simulink model "rev0BB"  (R2017b)
settings: Solver=FixedStepDiscrete  StartTime=0  StopTime=(((preLen+100+dataLenSymbols)*1+pad_first*3)*basePer)  RelTol=1e-3
values from neighbouring files (symbols this model uses):
  ack_stf_len_symbols = length(x_ACK_STF)    [rev0BB_setup.m]
  agc_delay_lag = 32    [rev0BB_setup.m]
  agc_detector_coef = ones(1,agc_detector_taps)./agc_detector_taps    [rev0BB_setup.m]
  agc_on = true    [rev0BB_startup.m]
  agc_sat_low = -agcSaturation    (= -12)    [rev0BB_setup.m]
  agc_sat_up = agcSaturation    (= 12)    [rev0BB_setup.m]
  agcDesired = 0    [rev0BB_setup.m]
  agcExpDomain = agcSaturation    (= 12)    [rev0BB_setup.m]
  agcExpResolution = 2^-5    (= 0.03125)    [rev0BB_setup.m]
  agcPwrAvgNum = 128    [rev0BB_setup.m]
  agcSaturation = 12    [rev0BB_setup.m]
  agcSettleThresh = 0.65    [rev0BB_setup.m]
  agcStep = 2^-8    (= 0.00390625)    [rev0BB_setup.m]
  atanDomain = 5    [rev0BB_setup.m]
  atanDomainTiming = 256    [rev0BB_setup.m]
  atanResolution = 2^-9    (= 0.001953125)    [rev0BB_setup.m]
  atanResolutionTiming = 2^-5    (= 0.03125)    [rev0BB_setup.m]
  averaging_num = ones(1, averaging_samples)    [rev0BB_setup.m]
  averaging_samples = 128    [rev0BB_setup.m]
  awgnSeed = abs(dBSnrRange(dBSnrInd)*1000+trial+10000000)    [plotBer.m]    (also in rev0BB_startup.m = 67)
  basePer = 1/baseFreq    (= 5e-08)    [rev0BB_setup.m]
  bitsPerSymbolHeader = log2(radixHeader)    [rev0BB_setup.m]
  bitsPerSymbolMax = log2(radixMax)    [rev0BB_setup.m]
  cal_sig_i_mult = 1.0    (= 1)    [rev0BB_startup.m]
  cal_sig_i_offset = 0.0    (= 0)    [rev0BB_startup.m]
  cal_sig_q_mult = 1.0    (= 1)    [rev0BB_startup.m]
  cal_sig_q_offset = 0.0    (= 0)    [rev0BB_startup.m]
  cefEarlyWarning = 256    [rev0BB_setup.m]
  cefLen = length(x_CEF)    [rev0BB_setup.m]
  channelFIR = zeros(1, round(maxSampleDelay)+1)    [rev0BB_startup.m]
  coarseCFOAdaptDelay = 1    [rev0BB_setup.m]
  cr_i = 0.020    (= 0.02)    [rev0BB_setup.m]
  cr_i_preamp = 2^-9    (= 0.001953125)    [rev0BB_setup.m]
  cr_int1_sat_low = -cr_integrator1_saturation    (= -0.6)    [rev0BB_setup.m]
  cr_int1_sat_up = cr_integrator1_saturation    (= 0.6)    [rev0BB_setup.m]
  cr_integrator1_decay = 1    [rev0BB_setup.m]
  cr_integrator1_saturation = 0.6    [rev0BB_setup.m]
  cr_mult_pipeline = 0    [rev0BB_setup.m]
  cr_p = 0.015    [rev0BB_setup.m]
  cr_sat2_low = -cr_saturation2    (= -0.6)    [rev0BB_setup.m]
  cr_sat2_up = cr_saturation2    (= 0.6)    [rev0BB_setup.m]
  cr_smooth_num = (1/cr_smooth_samples).*ones(1, cr_smooth_samples)    [rev0BB_setup.m]
  D_128 = [ 1,  8,  2,  4, 16, 32, 64]    [golay.m]    (also in rev0BB_setup.m)
  D_32 = [ 1,  4,  8,  2, 16]    [golay.m]    (also in rev0BB_setup.m)
  dataLenSymbols = header_len_bytes*8/bitsPerSymbolHeader + frame_len_bytes*8/bitsPerSymbol    [rev0BB_setup.m]
  default_channel = 3    [rev0BB_setup.m]
  dmm_coefs = ones(1,dmm_samples)./dmm_samples    [rev0BB_setup.m]
  dst_field_len = 8    [rev0BB_setup.m]
  expDomain = 3.3    [rev0BB_setup.m]
  expResolution = 2^-5    (= 0.03125)    [rev0BB_setup.m]
  expTol = .1    (= 0.1)    [rev0BB_setup.m]
  flush_delay = regular_pipeline*2+mult_pipeline+4    (= 4)    [rev0BB_setup.m]
  frac_lut_domain = 256    [rev0BB_setup.m]
  frac_lut_domain_cr = 64    [rev0BB_setup.m]
  frac_lut_range_max = 512    [rev0BB_setup.m]
  frac_lut_range_max_coarse_cfo = 127    [rev0BB_setup.m]
  frac_lut_range_max_cr = 127    [rev0BB_setup.m]
  frac_lut_range_min = -frac_lut_range_max    (= -512)    [rev0BB_setup.m]
  frac_lut_range_min_coarse_cfo = -frac_lut_range_max_coarse_cfo    (= -127)    [rev0BB_setup.m]
  frac_lut_range_min_cr = -frac_lut_range_max_cr    (= -127)    [rev0BB_setup.m]
  frac_lut_table_breaks = -frac_lut_domain:frac_lut_res:(frac_lut_domain-1)    [rev0BB_setup.m]
  frac_lut_table_breaks_coarse_cfo = -frac_lut_domain_coarse_cfo:frac_lut_res_coarse_cfo:(frac_lut_domain_coarse_cfo-1)    [rev0BB_setup.m]
  frac_lut_table_breaks_cr = -frac_lut_domain_cr:frac_lut_res_cr:(frac_lut_domain_cr-1)    [rev0BB_setup.m]
  frac_lut_table_data = 1./frac_lut_table_breaks    [rev0BB_setup.m]
  frac_lut_table_data_coarse_cfo = 1./frac_lut_table_breaks_coarse_cfo    [rev0BB_setup.m]
  frac_lut_table_data_cr = 1./frac_lut_table_breaks_cr    [rev0BB_setup.m]
  freeze_en_agc = true    [rev0BB_startup.m]
  freeze_en_cr_int1 = false    [rev0BB_startup.m]
  freeze_en_cr_int2 = false    [rev0BB_startup.m]
  freeze_en_cr_phase = false    [rev0BB_startup.m]
  freeze_en_tr_int1 = false    [rev0BB_startup.m]
  freeze_en_tr_int2 = false    [rev0BB_startup.m]
  freeze_en_tr_phase = false    [rev0BB_startup.m]
  freeze_on_cef_done = true    [rev0BB_startup.m]
  freeze_on_stf_done = false    [rev0BB_startup.m]
  freeze_on_valid = true    [rev0BB_startup.m]
  golay_type = 32    [rev0BB_setup.m]
  guardInt = int16(4)    [rev0BB_setup.m]
  guardTol = int16(5)    [rev0BB_setup.m]
  header_len_bytes = 8    [rev0BB_setup.m]
  lineWidth = 60    [rev0BB_setup.m]
  lmsEqDepth = 38    [rev0BB_setup.m]
  lmsStep_init = 0.006    [rev0BB_setup.m]
  lmsStep_meta = (lmsStep_final - lmsStep_init)/cefLen    [rev0BB_setup.m]
  lnDomain = 16    [rev0BB_setup.m]
  lnResolution = 2^-5    (= 0.03125)    [rev0BB_setup.m]
  local_node_id = 2    [rev0BB_startup.m]
  maxMsgSize = length(xSpectrum_PRE)+dataLenSymbols+300    [rev0BB_setup.m]
  minSTFPeaks = 3    [rev0BB_setup.m]
  mod_scheme_len_bytes = 1    [rev0BB_setup.m]
  modBPS = [1, 2, 4]    [rev0BB_setup.m]
  modKeys = [0, 1, 2]    [rev0BB_setup.m]
  mult_pipeline = 0    [rev0BB_setup.m]
  overSampleFreq = 80e6    (= 80000000)    [rev0BB_setup.m]
  overSamplePer = 1/overSampleFreq    (= 1.25e-08)    [rev0BB_setup.m]
  pad_first = 1000    [createTestVectors.m]
  post_cr_i_offset = 0    [rev0BB_startup.m]
  post_cr_q_offset = 0    [rev0BB_startup.m]
  preambleSequentialDetect = 2    [rev0BB_setup.m]
  preLen = length(x_PRE)    [rev0BB_setup.m]
  qam16_demod_scale_factor = qam16_hdl_distance/qam16_power_normalized_distance    [rev0BB_setup.m]
  rcRxFilt = [0.000303163120401141 -0.00118915940834234 -0.00187387637177 -0.00124167532697737 0.00029186889076529 0.00164526160586517 0.00182432050803312 0.000652133621739543 -0.00105668254004908 -0.00204011570659167 -0.00150058088768918 0.00026138356356816 0.0019831869994874 0.00231075800085521 0.000821993419120097 -0.00154687337975486 -0.00305430783933469 -0.00238186490079127 0.000301216962040692 0.00325307 ...(+2001 chars)    [rev0BB_setup.m]
  rcTxFilt = [0.000303163120401141 -0.00118915940834234 -0.00187387637177 -0.00124167532697737 0.00029186889076529 0.00164526160586517 0.00182432050803312 0.000652133621739543 -0.00105668254004908 -0.00204011570659167 -0.00150058088768918 0.00026138356356816 0.0019831869994874 0.00231075800085521 0.000821993419120097 -0.00154687337975486 -0.00305430783933469 -0.00238186490079127 0.000301216962040692 0.00325307 ...(+2001 chars)    [rev0BB_setup.m]
  regular_pipeline = 0    [rev0BB_setup.m]
  rx_gain = 1    [rev0BB_setup.m]
  rx_gain_i = 1    [rev0BB_setup.m]
  rx_gain_q = 1    [rev0BB_setup.m]
  rx_impare_i_offset = 0    [rev0BB_startup.m]
  rx_impare_i_scale = 1    [rev0BB_startup.m]
  rx_impare_q_offset = 0    [rev0BB_startup.m]
  rx_impare_q_scale = 1    [rev0BB_startup.m]
  rx_offset_correction_i = 0    [rev0BB_startup.m]
  rx_offset_correction_q = 0    [rev0BB_startup.m]
  sin_source_amp = 1    [rev0BB_setup.m]
  sin_source_freq = 250e6/16    (= 15625000)    [rev0BB_setup.m]
  slowPer = overSamplePer*slowSample    (= 2.5e-08)    [rev0BB_setup.m]
  std_pkt_type = 0    [rev0BB_setup.m]
  stfLen = length(x_STF)    [rev0BB_setup.m]
  testMsg = cat(1, xCTRL_PRE_adj, header, payload)    [plotBer.m]
  timing_i = 0.25    [rev0BB_setup.m]
  ... (+25 more)
undefined symbols (not defined in the file or in its folder): cr_integrator2_saturation, doppler, i, magnitude, useFadingChannel
libraries: helperLib x128, simulink x90, golayLib x34, dspsigops x32, commfilt2 x27, commdigbbndpm3 x8, hdlsllib x6, dsparch4 x4, commdigbbndam3 x4, commchan3 x2, commrflib2 x2, commcrc2 x2
(part 7 of 10)

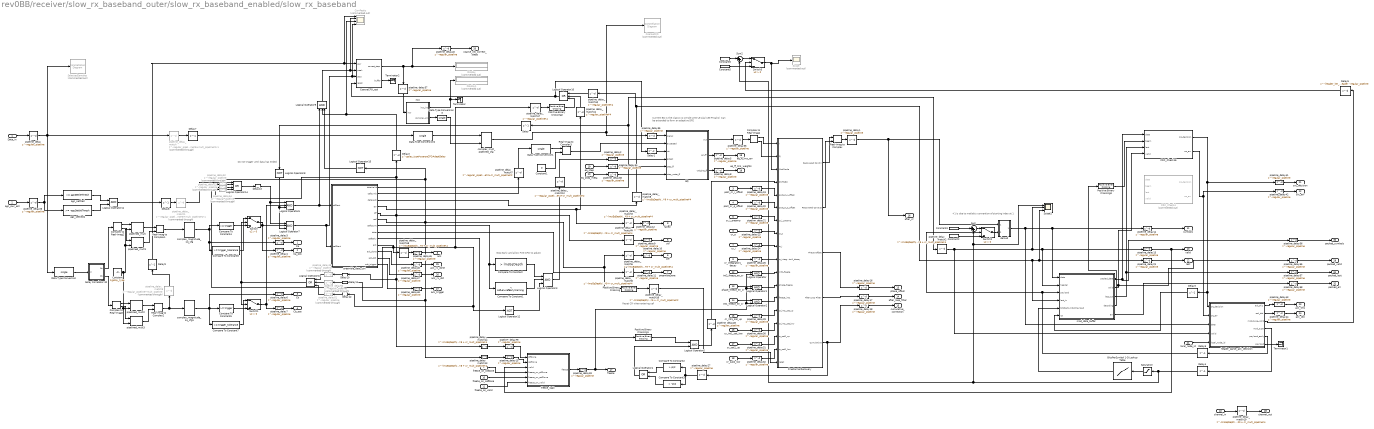
== system rev0BB/receiver/slow_rx_baseband_outer/slow_rx_baseband_enabled/slow_rx_baseband ==
  note: +1 is due to matlab's convention of starting index at 1
  note: Reset CR when entering cef
  note: Current EQ is the classic & simple LMS-LE Alg (see Proakis)
      | Can be extended to form an adaptive DFE
  note: Stop early and allow Fine CFO to adjust
  note: Do not trigger until data has ended
  Data_In : Inport  SampleTime=slowPer
  agc_pwr_est : Inport  Port=2  SampleTime=slowPer
  post_cr_i_offset : Inport  Port=3
  post_cr_q_offset : Inport  Port=4
  cr_i_preamp : Inport  Port=5
  cr_p : Inport  Port=6
  cr_i : Inport  Port=7
  cr_integrator1_decay : Inport  Port=8
  freeze_on_stfDone : Inport  Port=9
  freeze_on_cefDone : Inport  Port=10
  freeze_on_valid : Inport  Port=11
  int2_freeze_en_cr : Inport  Port=12  OutDataTypeStr=boolean
  phase_freeze_en_cr : Inport  Port=13  OutDataTypeStr=boolean
  int1_freeze_en_cr : Inport  Port=14  OutDataTypeStr=boolean
  cr_int1_sat_up : Inport  Port=15
  cr_int1_sat_low : Inport  Port=16
  cr_sat2_up : Inport  Port=17
  cr_sat2_low : Inport  Port=18
  eq_step : Inport  Port=19  OutDataTypeStr=fixdt(1,36,24)
  eq_step_meta : Inport  Port=20  OutDataTypeStr=fixdt(1,36,24)
  local_node_id : Inport  Port=21
  channel_in : Inport  Port=22  SampleTime=slowPer
  " BitsPerSymbol 1-D Lookup Table" : Lookup_n-D  NumberOfTableDimensions=1  BreakpointsForDimension1=modKeys  IndexSearchMethod=Evenly spaced points  Table=modBPS  InterpMethod=Flat  DiagnosticForOutOfRangeInput=Error  InternalRulePriority=Speed  RndMeth=Simplest  InputSameDT=on
  " CoarseCFO" : ConstellationDiagram  Commented=on
  " SelectedSamples" : ConstellationDiagram  Commented=on
  CRC_Check16 : Subsystem  TreatAsAtomicUnit=on
  CRC_Check4 : Subsystem  Commented=on
  CoarseCFO_est : Subsystem  TreatAsAtomicUnit=on
  Compare To Constant : simulink/Logic and Bit Operations/Compare To Constant  relop=>  const=lmsEqDepth  OutDataTypeStr=boolean
  Compare To Constant1 : simulink/Logic and Bit Operations/Compare To Constant  relop=<  const=cefLen-cefEarlyWarning  OutDataTypeStr=boolean
  Compare To Constant2 : simulink/Logic and Bit Operations/Compare To Constant  relop=>  const=pi/2  OutDataTypeStr=boolean
  Compare To Constant3 : simulink/Logic and Bit Operations/Compare To Constant  relop=<  const=-pi/2  OutDataTypeStr=boolean
  Compare To Constant4 : simulink/Logic and Bit Operations/Compare To Constant  relop=>=  const=trigger  OutDataTypeStr=boolean
  Compare To Constant5 : simulink/Logic and Bit Operations/Compare To Constant  relop=>=  const=trigger  OutDataTypeStr=boolean
  Compare To Constant6 : simulink/Logic and Bit Operations/Compare To Constant  relop=>=  const=trigger_tolerance  OutDataTypeStr=boolean
  Compare To Constant7 : simulink/Logic and Bit Operations/Compare To Constant  relop=>=  const=trigger_tolerance  OutDataTypeStr=boolean
  Complex to Real-Imag1 : ComplexToRealImag
  Complex to Real-Imag2 : ComplexToRealImag
  Complex to Real-Imag3 : ComplexToRealImag
  Constant : Constant  Value=1/golay_type  OutDataTypeStr=Inherit: Inherit via back propagation  SampleTime=-1
  Constant1 : Constant  Value=0  OutDataTypeStr=Inherit: Inherit via back propagation  SampleTime=-1
  Constant{2..3,5..6} (4 alike) : Constant  OutDataTypeStr=uint8  SampleTime=-1
  CorrPeaks : Scope  Commented=on  NumInputPorts=4
  Data Type Conversion{,1..3} (4 alike) : DataTypeConversion  OutDataTypeStr=single
  Delay : Delay  DelayLength=1  InitialCondition=0
  Delay1 : Delay  InitialCondition=0
  Delay{3..5,7..13} (10 alike) : Delay  DelayLength=1
  Delay2 : Delay  DelayLength=golay_type*coarseCFOAdaptDelay
  Delay6 : Delay  DelayLength=(header_len_bytes-mod_scheme_len_bytes)*8/bitsPerSymbolHeader - regular_pipeline
  Display : Display  Commented=on
  Display1 : Display  Commented=on
  EQ : Subsystem  TreatAsAtomicUnit=on
  FineCarrierRecovery : Subsystem  RequirementInfo={} %GIDa_d02aedaf_4fff_4ad7_becd_06d8542c600d  TreatAsAtomicUnit=on
  Golay Correlator 32 : Subsystem  TreatAsAtomicUnit=on
  Logical Operator{,1..2,5,11} (5 alike) : Logic  AllPortsSameDT=off  OutDataTypeStr=boolean
  Logical Operator10 : Logic  Operator=OR  Inputs=3  AllPortsSameDT=off  OutDataTypeStr=boolean
  Logical Operator12 : Logic  Operator=NOT  AllPortsSameDT=off  OutDataTypeStr=boolean
  Logical Operator13 : Logic  Operator=OR  Inputs=3  AllPortsSameDT=off  OutDataTypeStr=boolean
  Logical Operator14 : Logic  Operator=OR  Inputs=4  AllPortsSameDT=off  OutDataTypeStr=boolean
  Logical Operator15 : Logic  Operator=NOT  AllPortsSameDT=off  OutDataTypeStr=boolean
  Logical Operator{3,6..7,9} (4 alike) : Logic  Inputs=3  AllPortsSameDT=off  OutDataTypeStr=boolean
  Logical Operator4 : Logic  Operator=OR  AllPortsSameDT=off  OutDataTypeStr=boolean
  Logical Operator8 : Logic  Operator=NOT  AllPortsSameDT=off  OutDataTypeStr=boolean
  Positive Binary Crossing{,1..3} (4 alike) : helperLib/Positive Binary Crossing
  Real-Imag to Complex{,1..3} (4 alike) : RealImagToComplex
  Saturation : Saturate  UpperLimit=modKeys(length(modKeys))  LowerLimit=modKeys(1)
  Scope : Scope  Commented=on
  Scope1 : Scope  NumInputPorts=3
  Sum : Sum  Inputs=|++  OutDataTypeStr=Inherit: Inherit via back propagation
  Sum2 : Sum  Inputs=|++  OutDataTypeStr=Inherit: Inherit via back propagation
  Switch{,1..3} (4 alike) : Switch  Criteria=u2 > Threshold
  Terminator : Terminator
  Terminator1 : Terminator
  Terminator2 : Terminator
  agc_settled : simulink/Logic and Bit Operations/Compare To Constant  relop=<=  const=agcSettleThresh  OutDataTypeStr=boolean
  agc_settled1 : simulink/Logic and Bit Operations/Compare To Constant  relop=>=  const=-agcSettleThresh  OutDataTypeStr=boolean
  complex_magnitude_sq_cfg : helperLib/complex_magnitude_sq_cfg  mult=mult_pipeline  pipe=regular_pipeline
  complex_magnitude_sq_cfg1 : helperLib/complex_magnitude_sq_cfg  mult=mult_pipeline  pipe=regular_pipeline
  complex_mult_pipelined_cfg : helperLib/complex_mult_pipelined_cfg  mult=cr_mult_pipeline  pipe=regular_pipeline
  demod : Subsystem
  freeze_logic : Subsystem  TreatAsAtomicUnit=on
  header_parse_ack_decision : Subsystem  TreatAsAtomicUnit=on
  mod_data_buffer : Subsystem  TreatAsAtomicUnit=on
  nco : Subsystem  TreatAsAtomicUnit=on
  pipeline_delay{,1..48,55..58} (53 alike) : Delay  DelayLength=regular_pipeline
  pipeline_delay{49..54} (6 alike) : Delay  Commented=through  DelayLength=regular_pipeline
  pipeline_delay_match : Delay  Commented=through  DelayLength=regular_pipeline*8+mult_pipeline*2-1
  pipeline_delay_match1 : Delay  Commented=through  DelayLength=regular_pipeline*8+mult_pipeline*2-1
  pipeline_delay_match10 : Delay  DelayLength=regular_pipeline*4
  pipeline_delay_match11 : Delay  DelayLength=regular_pipeline*4
  pipeline_delay_match12 : Delay  DelayLength=regular_pipeline*2+cr_mult_pipeline*2
  pipeline_delay_match13 : Delay  DelayLength=lmsEqDepth/2-1 + regular_pipeline*8 + cr_mult_pipeline*4
  pipeline_delay_match14 : Delay  DelayLength=lmsEqDepth/2-1 + regular_pipeline*8 + cr_mult_pipeline*4
  pipeline_delay_match16 : Delay  DelayLength=lmsEqDepth/2-1 + regular_pipeline*5 + cr_mult_pipeline*2
  pipeline_delay_match17 : Delay  DelayLength=regular_pipeline*4
  pipeline_delay_match{2..6,8,18} (7 alike) : Delay  DelayLength=lmsEqDepth/2-1 + regular_pipeline*9 + cr_mult_pipeline*4
  pipeline_delay_match19 : Delay  DelayLength=lmsEqDepth + regular_pipeline*20 + cr_mult_pipeline*4
  pipeline_delay_match7 : Delay  DelayLength=regular_pipeline*2+cr_mult_pipeline*2
  pipeline_delay_match9 : Delay  Commented=through  DelayLength=regular_pipeline+mult_pipeline
  pipelined_mult{,1..3} (4 alike) : helperLib/pipelined_mult  d=mult_pipeline
  preamble_data_ctrl : Subsystem  TreatAsAtomicUnit=on
  Ca : Outport  SampleTime=slowPer
  Ca_pos : Outport  Port=2  SampleTime=slowPer
  Cb : Outport  Port=3  SampleTime=slowPer
  Cb_pos : Outport  Port=4  SampleTime=slowPer
  stf : Outport  Port=5  SampleTime=slowPer
  cef : Outport  Port=6  SampleTime=slowPer
  preambleDone : Outport  Port=7  SampleTime=slowPer
  ack : Outport  Port=8  SampleTime=slowPer
  failed : Outport  Port=9  SampleTime=slowPer
  valid : Outport  Port=10  SampleTime=slowPer
  symbols : Outport  Port=11  SampleTime=slowPer
  last : Outport  Port=12  SampleTime=slowPer
  phase_offset : Outport  Port=13  SampleTime=slowPer
  after_loop_filter : Outport  Port=14  SampleTime=slowPer
  cumulative_correction : Outport  Port=15  SampleTime=slowPer
  after_cr : Outport  Port=16  SampleTime=slowPer
  freeze : Outport  Port=17  SampleTime=slowPer
  eq_ff_lms_err : Outport  Port=18  SampleTime=slowPer
  eq_ff_lms_weights : Outport  Port=19  SampleTime=slowPer
  coarse_cfo_correct_steps : Outport  Port=20  SampleTime=slowPer
  crc_decision : Outport  Port=21  SampleTime=slowPer
  crc_err : Outport  Port=22  SampleTime=slowPer
  ack_this : Outport  Port=23  SampleTime=slowPer
  ack_dst : Outport  Port=24  SampleTime=slowPer
  ack_rx_done : Outport  Port=25  SampleTime=slowPer
  ack_rx_dst : Outport  Port=26  SampleTime=slowPer
  ack_trigger : Outport  Port=27
  channel_out : Outport  Port=28  SampleTime=slowPer
  packed_valid : Outport  Port=29  SampleTime=slowPer
  packed_symbols : Outport  Port=30  SampleTime=slowPer
  packed_last : Outport  Port=31  SampleTime=slowPer
  packed_err : Outport  Port=32  SampleTime=slowPer
  wires:
  Complex to Real-Imag1/1 -> FineCarrierRecovery/1(I)
  Complex to Real-Imag1/2 -> FineCarrierRecovery/2(Q)
  FineCarrierRecovery/1(Recovered Const I) -> Real-Imag to Complex/1
  FineCarrierRecovery/2(Recovered Const Q) -> Real-Imag to Complex/2
  FineCarrierRecovery/3(Phase Offset) -> pipeline_delay16/1
  FineCarrierRecovery/4(After Loop Filter) -> pipeline_delay17/1
  FineCarrierRecovery/5(Cumulative) -> pipeline_delay27/1, pipeline_delay18/1
  pipeline_delay14/1 -> symbols/1
  pipeline_delay13/1 -> freeze_logic/3(valid), valid/1
  pipeline_delay12/1 -> failed/1
  pipeline_delay11/1 -> preambleDone/1
  pipeline_delay10/1 -> cef/1
  pipeline_delay9/1 -> stf/1
  pipeline_delay7/1 -> Cb_pos/1
  pipeline_delay6/1 -> Cb/1
  pipeline_delay4/1 -> Ca_pos/1
  pipeline_delay3/1 -> Ca/1
  Real-Imag to Complex/1 -> pipeline_delay1/1
  Data_In/1 -> pipeline_delay/1
  pipeline_delay16/1 -> phase_offset/1
  pipeline_delay17/1 -> after_loop_filter/1
  pipeline_delay18/1 -> cumulative_correction/1
  post_cr_i_offset/1 -> pipeline_delay19/1
  post_cr_q_offset/1 -> pipeline_delay20/1
  pipeline_delay19/1 -> FineCarrierRecovery/5(post_cr_i_offset)
  pipeline_delay20/1 -> FineCarrierRecovery/6(post_cr_q_offset)
  cr_i_preamp/1 -> pipeline_delay22/1
  cr_p/1 -> pipeline_delay23/1
  cr_i/1 -> pipeline_delay24/1
  cr_integrator1_decay/1 -> pipeline_delay25/1
  pipeline_delay22/1 -> FineCarrierRecovery/7(cr_i_preamp)
  pipeline_delay23/1 -> FineCarrierRecovery/8(cr_p)
  pipeline_delay24/1 -> FineCarrierRecovery/9(cr_i)
  pipeline_delay25/1 -> FineCarrierRecovery/10(cr_integrator1_decay)
  pipeline_delay33/1 -> Logical Operator2/2, Logical Operator1/2, Logical Operator/2, freeze/1
  freeze_on_stfDone/1 -> freeze_logic/4(freeze_on_stfDone)
  freeze_on_cefDone/1 -> freeze_logic/5(freeze_on_cefDone)
  freeze_on_valid/1 -> freeze_logic/6(freeze_on_valid)
  freeze_logic/1(freeze) -> pipeline_delay33/1
  Logical Operator/1 -> FineCarrierRecovery/11(int2_freeze)
  int2_freeze_en_cr/1 -> Logical Operator/1
  cr_int1_sat_up/1 -> pipeline_delay29/1
  pipeline_delay29/1 -> FineCarrierRecovery/14(cr_int1_sat_up)
  cr_sat2_low/1 -> pipeline_delay32/1
  pipeline_delay32/1 -> FineCarrierRecovery/17(cr_sat2_low)
  cr_sat2_up/1 -> pipeline_delay31/1
  pipeline_delay31/1 -> FineCarrierRecovery/16(cr_sat2_up)
  cr_int1_sat_low/1 -> pipeline_delay30/1
  pipeline_delay30/1 -> FineCarrierRecovery/15(cr_int1_sat_low)
  phase_freeze_en_cr/1 -> Logical Operator1/1
  Logical Operator1/1 -> FineCarrierRecovery/12(phase_freeze)
  Logical Operator2/1 -> FineCarrierRecovery/13(freeze_int1)
  int1_freeze_en_cr/1 -> Logical Operator2/1
  pipeline_delay21/1 -> last/1
  Real-Imag to Complex1/1 -> complex_magnitude_sq_cfg/1
  Golay Correlator 32/1(Ca) -> Complex to Real-Imag2/1
  Complex to Real-Imag2/1 -> pipelined_mult/1
  Complex to Real-Imag2/2 -> pipelined_mult1/1
  pipelined_mult/1 -> Real-Imag to Complex1/1
  pipelined_mult1/1 -> Real-Imag to Complex1/2
  Constant/1 -> pipelined_mult1/2, pipelined_mult/2, pipelined_mult3/2, pipelined_mult2/2
  Complex to Real-Imag3/1 -> pipelined_mult2/1
  Complex to Real-Imag3/2 -> pipelined_mult3/1
  pipelined_mult2/1 -> Real-Imag to Complex2/1
  pipelined_mult3/1 -> Real-Imag to Complex2/2
  Golay Correlator 32/2(Cb) -> Complex to Real-Imag3/1
  Data Type Conversion/1 -> Golay Correlator 32/1(In)
  agc_pwr_est/1 -> pipeline_delay26/1
  pipeline_delay26/1 -> agc_settled/1, agc_settled1/1
  Logical Operator6/1 -> preamble_data_ctrl/1(stfStart), Logical Operator9/1
  Logical Operator7/1 -> CorrPeaks/4, CoarseCFO_est/3(stop), preamble_data_ctrl/2(cefStart)
  Logical Operator11/1 -> Delay8/1
  Data Type Conversion1/1 -> Real-Imag to Complex3/1
  Constant1/1 -> Real-Imag to Complex3/2
  pipeline_delay_match/1 -> Delay7/1
  Compare To Constant/1 -> Logical Operator3/1
  Compare To Constant1/1 -> Logical Operator3/2
  Logical Operator3/1 -> pipeline_delay_match12/1
  Compare To Constant2/1 -> Logical Operator4/1
  Compare To Constant3/1 -> Logical Operator4/2
  pipeline_delay27/1 -> Compare To Constant3/1, Compare To Constant2/1
  Logical Operator4/1 -> Logical Operator5/2
  Positive Binary Crossing1/1 -> Logical Operator5/1
  Logical Operator5/1 -> pipeline_delay28/1
  pipeline_delay28/1 -> FineCarrierRecovery/4(Shift180)
  demod/1(Out1) -> pipeline_delay14/1, mod_data_buffer/1(data), header_parse_ack_decision/3(data)
  pipeline_delay_match3/1 -> pipeline_delay12/1
  pipeline_delay_match6/1 -> pipeline_delay11/1
  pipeline_delay_match5/1 -> pipeline_delay10/1
  pipeline_delay_match4/1 -> pipeline_delay9/1
  Logical Operator8/1 -> Logical Operator6/3, Logical Operator7/3
  Delay/1 -> Logical Operator8/1
  eq_step/1 -> pipeline_delay34/1
  pipeline_delay/1 -> Data Type Conversion/1, " SelectedSamples"/1, pipeline_delay_match/1
  pipeline_delay36/1 -> Complex to Real-Imag1/1
  Real-Imag to Complex2/1 -> complex_magnitude_sq_cfg1/1, pipeline_delay_match9/1
  Logical Operator9/1 -> CoarseCFO_est/2(peak), CorrPeaks/2
  pipeline_delay_match10/1 -> Logical Operator10/1
  Logical Operator10/1 -> CoarseCFO_est/4(reset), Delay1/1
  pipeline_delay_match9/1 -> Delay9/1
  CoarseCFO_est/1(correct_step) -> Display/1, pipeline_delay40/1, pipeline_delay37/1
  complex_mult_pipelined_cfg/1 -> pipeline_delay35/1, " CoarseCFO"/1
  pipeline_delay_match11/1 -> Logical Operator10/2
  pipeline_delay_match7/1 -> Data Type Conversion1/1
  Real-Imag to Complex3/1 -> EQ/2(expected)
  Delay1/1 -> EQ/3(rst)
  pipeline_delay_match12/1 -> pipeline_delay2/1
  pipeline_delay34/1 -> EQ/5(step_ff)
  EQ/1(out) -> pipeline_delay36/1
  EQ/2(err_ff) -> pipeline_delay5/1
  pipeline_delay35/1 -> EQ/1(signal)
  agc_settled/1 -> Logical Operator11/1
  agc_settled1/1 -> Logical Operator11/2
  eq_step_meta/1 -> pipeline_delay38/1
  pipeline_delay38/1 -> EQ/6(step_meta_ff)
  pipeline_delay_match13/1 -> pipeline_delay15/1
  pipeline_delay_match14/1 -> pipeline_delay39/1
  pipeline_delay15/1 -> freeze_logic/2(cefDone)
  pipeline_delay39/1 -> freeze_logic/1(stfDone)
  pipeline_delay5/1 -> eq_ff_lms_err/1
  EQ/3(weights_ff) -> pipeline_delay8/1
  pipeline_delay8/1 -> eq_ff_lms_weights/1
  pipeline_delay40/1 -> coarse_cfo_correct_steps/1
  CoarseCFO_est/2(buffer) -> Terminator2/1
  preamble_data_ctrl/6(cef) -> Logical Operator15/1, pipeline_delay53/1, Delay11/1, pipeline_delay_match13/1, Positive Binary Crossing/1, pipeline_delay_match5/1
  preamble_data_ctrl/4(err) -> pipeline_delay_match3/1, pipeline_delay_match11/1
  preamble_data_ctrl/7(cefCount) -> Compare To Constant/1, Compare To Constant1/1
  preamble_data_ctrl/2(cefSymb) -> pipeline_delay_match7/1
  preamble_data_ctrl/3(dataLast) -> pipeline_delay_match8/1
  preamble_data_ctrl/8(data) -> pipeline_delay_match6/1
  preamble_data_ctrl/9(cefEarly) -> Positive Binary Crossing1/1
  pipeline_delay37/1 -> nco/1(incr)
  nco/1(incr_int) -> Terminator/1, Display1/1
  Positive Binary Crossing/1 -> pipeline_delay_match16/1
  pipeline_delay_match16/1 -> FineCarrierRecovery/18(reset)
  pipeline_delay41/1 -> crc_decision/1
  pipeline_delay42/1 -> crc_err/1
  CRC_Check16/2(crc_err) -> pipeline_delay42/1, header_parse_ack_decision/2(crc_err)
  CRC_Check16/1(crc_decision) -> pipeline_delay41/1, header_parse_ack_decision/1(crc_decision), Delay3/1
  local_node_id/1 -> header_parse_ack_decision/5(local_node_id)
  header_parse_ack_decision/1(ack_this) -> pipeline_delay43/1
  header_parse_ack_decision/2(ack_dst) -> pipeline_delay44/1
  pipeline_delay43/1 -> ack_this/1
  pipeline_delay44/1 -> ack_dst/1
  Logical Operator12/1 -> Logical Operator3/3
  Positive Binary Crossing2/1 -> Logical Operator10/3
  pipeline_delay_match17/1 -> Positive Binary Crossing2/1
  preamble_data_ctrl/10(ack) -> pipeline_delay54/1, pipeline_delay_match18/1, pipeline_delay_match17/1, Delay12/1, Logical Operator12/1
  pipeline_delay45/1 -> ack/1
  pipeline_delay46/1 -> ack_rx_done/1
  pipeline_delay47/1 -> ack_rx_dst/1
  preamble_data_ctrl/11(ack_done) -> pipeline_delay46/1
  preamble_data_ctrl/12(ack_dst) -> pipeline_delay47/1
  pipeline_delay_match18/1 -> pipeline_delay45/1
  pipeline_delay48/1 -> ack_trigger/1
  preamble_data_ctrl/13(ack_trigger) -> pipeline_delay48/1
  Logical Operator14/1 -> Delay13/1
  channel_in/1 -> pipeline_delay_match19/1
  pipeline_delay_match19/1 -> channel_out/1
  pipeline_delay2/1 -> EQ/4(adapt)
  complex_magnitude_sq_cfg/1 -> Compare To Constant4/1, Compare To Constant6/1, pipeline_delay3/1
  Switch/1 -> pipeline_delay4/1, Logical Operator7/2
  complex_magnitude_sq_cfg1/1 -> Compare To Constant7/1, Compare To Constant5/1, pipeline_delay6/1
  Switch1/1 -> pipeline_delay7/1, Logical Operator6/2
  Compare To Constant4/1 -> Switch/3
  Compare To Constant5/1 -> Switch1/3
  Compare To Constant7/1 -> Switch1/1
  Compare To Constant6/1 -> Switch/1
  Logical Operator13/1 -> Switch/2, Switch1/2
  pipeline_delay49/1 -> Logical Operator13/1
  pipeline_delay50/1 -> Logical Operator13/2
  pipeline_delay51/1 -> Logical Operator13/3
  pipeline_delay_match1/1 -> Logical Operator14/1
  pipeline_delay52/1 -> Logical Operator14/2
  pipeline_delay53/1 -> Logical Operator14/3
  pipeline_delay54/1 -> Logical Operator14/4
  Data Type Conversion2/1 -> complex_mult_pipelined_cfg/1
  nco/2(complex_sin) -> Data Type Conversion3/1
  preamble_data_ctrl/5(stf) -> Delay10/1, pipeline_delay_match14/1, pipeline_delay_match4/1, Delay2/1, pipeline_delay52/1
  Delay2/1 -> CorrPeaks/3, Logical Operator9/2
  Logical Operator15/1 -> Logical Operator9/3
  pipeline_delay_match2/1 -> Scope1/2, mod_data_buffer/2(header), pipeline_delay13/1, header_parse_ack_decision/4(valid)
  Switch3/1 -> Scope/1, FineCarrierRecovery/3(ModMode)
  header_parse_ack_decision/5(payload_early) -> Delay5/1
  header_parse_ack_decision/4(mod_type) -> Delay4/1
  Saturation/1 -> " BitsPerSymbol 1-D Lookup Table"/1
  " BitsPerSymbol 1-D Lookup Table"/1 -> mod_data_buffer/5(bitsPerSymbolPayload)
  Switch2/1 -> demod/2(ModMode)
  Constant2/1 -> Switch2/3
  Sum/1 -> Switch2/1
  Constant3/1 -> Sum/1
  Sum2/1 -> Switch3/1
  Constant6/1 -> Sum2/1
  Constant5/1 -> Switch3/3
  Delay3/1 -> mod_data_buffer/6(rst)
  mod_data_buffer/1(packed_data) -> CRC_Check16/1(data), pipeline_delay56/1
  mod_data_buffer/2(valid) -> CRC_Check16/4(valid), pipeline_delay55/1
  pipeline_delay56/1 -> packed_symbols/1
  pipeline_delay55/1 -> packed_valid/1
  pipeline_delay57/1 -> packed_last/1
  mod_data_buffer/3(last_out) -> CRC_Check16/3(last), pipeline_delay57/1
  pipeline_delay_match8/1 -> mod_data_buffer/4(last_in), Scope1/3, pipeline_delay21/1, pipeline_delay_match10/1
  preamble_data_ctrl/1(dataValid) -> Delay/1, pipeline_delay_match2/1
  pipeline_delay1/1 -> after_cr/1, demod/1(In1)
  Delay4/1 -> Scope1/1, Sum/2, Sum2/2, Saturation/1
  Delay5/1 -> mod_data_buffer/3(payload), Switch2/2
  header_parse_ack_decision/6(payload) -> Terminator1/1
  header_parse_ack_decision/3(mod_type_valid) -> Delay6/1
  Delay6/1 -> Switch3/2
  Positive Binary Crossing3/1 -> CRC_Check16/2(begin)
  mod_data_buffer/4(decoding) -> Positive Binary Crossing3/1
  pipeline_delay58/1 -> packed_err/1
  mod_data_buffer/5(err) -> pipeline_delay58/1
  Data Type Conversion3/1 -> complex_mult_pipelined_cfg/2
  Delay7/1 -> Data Type Conversion2/1
  Delay8/1 -> pipeline_delay_match1/1
  Delay9/1 -> CoarseCFO_est/1(corr), CorrPeaks/1
  Delay10/1 -> pipeline_delay49/1
  Delay11/1 -> pipeline_delay50/1
  Delay12/1 -> pipeline_delay51/1
  Delay13/1 -> Logical Operator7/1, Logical Operator6/1

== system rev0BB/receiver/fast_rx_baseband/Timing Recovery/loopFilter/sat ==
  In1 : Inport
  limit_up : Inport  Port=2
  limit_low : Inport  Port=3
  Saturation : Saturate  Commented=on  UpperLimit=timing_integrate1_saturate  LowerLimit=-timing_integrate1_saturate
  Saturation Dynamic : simulink/Discontinuities/Saturation Dynamic  OutMin=[]  OutMax=[]  OutDataTypeStr=Inherit: Same as second input  OutDataType=fixdt(1, 16)  OutScaling=2^-10  DoSatur=off
  pipeline_delay : Delay  DelayLength=regular_pipeline
  Out1 : Outport
  wires:
  In1/1 -> pipeline_delay/1
  limit_up/1 -> Saturation Dynamic/1
  limit_low/1 -> Saturation Dynamic/3
  pipeline_delay/1 -> Saturation Dynamic/2
  Saturation Dynamic/1 -> Out1/1

== system rev0BB/receiver/fast_rx_baseband/Timing Recovery/loopFilter/sat1 ==
  In1 : Inport
  limit_up : Inport  Port=2
  limit_low : Inport  Port=3
  Saturation : Saturate  Commented=on  UpperLimit=timing_integrate1_saturate  LowerLimit=-timing_integrate1_saturate
  Saturation Dynamic : simulink/Discontinuities/Saturation Dynamic  OutMin=[]  OutMax=[]  OutDataTypeStr=Inherit: Same as second input  OutDataType=fixdt(1, 16)  OutScaling=2^-10  DoSatur=off
  pipeline_delay : Delay  DelayLength=regular_pipeline
  Out1 : Outport
  wires:
  In1/1 -> pipeline_delay/1
  limit_up/1 -> Saturation Dynamic/1
  limit_low/1 -> Saturation Dynamic/3
  pipeline_delay/1 -> Saturation Dynamic/2
  Saturation Dynamic/1 -> Out1/1

== system rev0BB/receiver/fast_rx_baseband/Timing Recovery/nda_4x_time_err_enable/phase_est ==
  In1 : Inport
  In2 : Inport  Port=2
  In3 : Inport  Port=3
  In4 : Inport  Port=4
  Enable : EnablePort
  complex_magnitude_sq_cfg{,1..3} (4 alike) : helperLib/complex_magnitude_sq_cfg  mult=wide_mult_pipeline  pipe=regular_pipeline
  pipeline_delay{1..3,8} (4 alike) : Delay  DelayLength=regular_pipeline
  timing_rec_sym_rate_enb : Subsystem
  Out1 : Outport  InitialOutput=[0]
  wires:
  In1/1 -> pipeline_delay1/1
  timing_rec_sym_rate_enb/1(err) -> Out1/1
  complex_magnitude_sq_cfg/1 -> timing_rec_sym_rate_enb/1(delay3)
  complex_magnitude_sq_cfg1/1 -> timing_rec_sym_rate_enb/2(delay2)
  complex_magnitude_sq_cfg2/1 -> timing_rec_sym_rate_enb/3(delay1)
  complex_magnitude_sq_cfg3/1 -> timing_rec_sym_rate_enb/4(delay0)
  In2/1 -> pipeline_delay2/1
  In3/1 -> pipeline_delay3/1
  In4/1 -> pipeline_delay8/1
  pipeline_delay3/1 -> complex_magnitude_sq_cfg2/1
  pipeline_delay1/1 -> complex_magnitude_sq_cfg/1
  pipeline_delay2/1 -> complex_magnitude_sq_cfg1/1
  pipeline_delay8/1 -> complex_magnitude_sq_cfg3/1

== system rev0BB/receiver/fast_rx_baseband/Timing Recovery/nda_4x_time_err_enable/tapped_delay4  ==
  symbol : Inport
  Delay : Delay  DelayLength=1  InitialCondition=0
  Delay1 : Delay  DelayLength=1  InitialCondition=0
  Delay2 : Delay  DelayLength=1  InitialCondition=0
  delay_3 : Outport
  delay_2 : Outport  Port=2
  delay_1 : Outport  Port=3
  delay_0 : Outport  Port=4
  wires:
  Delay2/1 -> delay_3/1
  Delay1/1 -> delay_2/1, Delay2/1
  Delay/1 -> delay_1/1, Delay1/1
  symbol/1 -> delay_0/1, Delay/1

== system rev0BB/receiver/slow_rx_baseband_outer/slow_rx_baseband_enabled/slow_rx_baseband/CRC_Check16 ==
  note: Entire frame will be forwarded to the host, including the CRC check.  Due to the latency of the CRC check,
      | we will not know if the CRC has passed until after the entire packet has been sent to the host.
  data : Inport
  begin : Inport  Port=2
  last : Inport  Port=3
  valid : Inport  Port=4
  Data Type Conversion : DataTypeConversion  OutDataTypeStr=fixdt(0,4,0)
  Data Type Conversion{1..4} (4 alike) : DataTypeConversion  OutDataTypeStr=uint8
  Extract Bits : simulink/Logic and Bit Operations/Extract Bits  bitsToExtract=Range of bits  numBits=8  bitIdxRange=[0 0]  outScalingMode=Treat bit field as an integer
      settings: SourceProductName=Simulink
  Extract Bits1 : simulink/Logic and Bit Operations/Extract Bits  bitsToExtract=Range of bits  numBits=8  bitIdxRange=[1 1]  outScalingMode=Treat bit field as an integer
      settings: SourceProductName=Simulink
  Extract Bits2 : simulink/Logic and Bit Operations/Extract Bits  bitsToExtract=Range of bits  numBits=8  bitIdxRange=[2 2]  outScalingMode=Treat bit field as an integer
      settings: SourceProductName=Simulink
  Extract Bits3 : simulink/Logic and Bit Operations/Extract Bits  bitsToExtract=Range of bits  numBits=8  bitIdxRange=[3 3]  outScalingMode=Treat bit field as an integer
      settings: SourceProductName=Simulink
  Gain : Gain  Gain=8
  Gain1 : Gain  Gain=4
  Gain2 : Gain  Gain=2
  General CRC Syndrome Detector HDL Optimized : commcrc2/General CRC Syndrome Detector HDL Optimized  Polynomial=crc_poly  InitialState=crc_init  DirectMethod=off  ReflectInput=off  ReflectCRCChecksum=off  FinalXORValue=crc_xor  SimulateUsing=Code generation
      settings: SourceProductName=Communications System Toolbox  SourceProductBaseCode=CM
  Logical Operator12 : Logic  AllPortsSameDT=off  OutDataTypeStr=boolean
  Sum : Sum  Inputs=|++++  OutDataTypeStr=Inherit: Same as first input
  Terminator1 : Terminator
  Terminator2 : Terminator
  crc_decision : Outport
  crc_err : Outport  Port=2
  wires:
  valid/1 -> General CRC Syndrome Detector HDL Optimized/4
  General CRC Syndrome Detector HDL Optimized/2 -> Terminator1/1
  General CRC Syndrome Detector HDL Optimized/3 -> Logical Operator12/1
  Logical Operator12/1 -> crc_decision/1
  General CRC Syndrome Detector HDL Optimized/5 -> crc_err/1
  General CRC Syndrome Detector HDL Optimized/4 -> Logical Operator12/2
  begin/1 -> General CRC Syndrome Detector HDL Optimized/2
  last/1 -> General CRC Syndrome Detector HDL Optimized/3
  Extract Bits1/1 -> Data Type Conversion4/1
  Extract Bits/1 -> Data Type Conversion1/1
  General CRC Syndrome Detector HDL Optimized/1 -> Terminator2/1
  Data Type Conversion/1 -> General CRC Syndrome Detector HDL Optimized/1
  data/1 -> Extract Bits3/1, Extract Bits2/1, Extract Bits1/1, Extract Bits/1
  Data Type Conversion1/1 -> Gain/1
  Data Type Conversion4/1 -> Gain1/1
  Sum/1 -> Data Type Conversion/1
  Gain/1 -> Sum/1
  Extract Bits2/1 -> Data Type Conversion2/1
  Extract Bits3/1 -> Data Type Conversion3/1
  Gain1/1 -> Sum/2
  Data Type Conversion2/1 -> Gain2/1
  Gain2/1 -> Sum/3
  Data Type Conversion3/1 -> Sum/4

== system rev0BB/receiver/slow_rx_baseband_outer/slow_rx_baseband_enabled/slow_rx_baseband/CRC_Check4 ==
  note: Entire frame will be forwarded to the host, including the CRC check.  Due to the latency of the CRC check,
      | we will not know if the CRC has passed until after the entire packet has been sent to the host.
  data : Inport
  begin : Inport  Port=2
  last : Inport  Port=3
  valid : Inport  Port=4
  Data Type Conversion : DataTypeConversion  OutDataTypeStr=fixdt(0,2,0)
  Data Type Conversion1 : DataTypeConversion  OutDataTypeStr=uint8
  Data Type Conversion4 : DataTypeConversion  OutDataTypeStr=uint8
  Extract Bits : simulink/Logic and Bit Operations/Extract Bits  bitsToExtract=Range of bits  numBits=8  bitIdxRange=[0 0]  outScalingMode=Treat bit field as an integer
      settings: SourceProductName=Simulink
  Extract Bits1 : simulink/Logic and Bit Operations/Extract Bits  bitsToExtract=Range of bits  numBits=8  bitIdxRange=[1 1]  outScalingMode=Treat bit field as an integer
      settings: SourceProductName=Simulink
  Gain : Gain  Gain=2
  General CRC Syndrome Detector HDL Optimized : commcrc2/General CRC Syndrome Detector HDL Optimized  Polynomial=crc_poly  InitialState=crc_init  DirectMethod=off  ReflectInput=off  ReflectCRCChecksum=off  FinalXORValue=crc_xor  SimulateUsing=Code generation
      settings: SourceProductName=Communications System Toolbox  SourceProductBaseCode=CM
  Logical Operator12 : Logic  AllPortsSameDT=off  OutDataTypeStr=boolean
  Sum : Sum  Inputs=|++  OutDataTypeStr=Inherit: Same as first input
  Terminator1 : Terminator
  Terminator2 : Terminator
  crc_decision : Outport
  crc_err : Outport  Port=2
  wires:
  valid/1 -> General CRC Syndrome Detector HDL Optimized/4
  General CRC Syndrome Detector HDL Optimized/2 -> Terminator1/1
  General CRC Syndrome Detector HDL Optimized/3 -> Logical Operator12/1
  Logical Operator12/1 -> crc_decision/1
  General CRC Syndrome Detector HDL Optimized/5 -> crc_err/1
  General CRC Syndrome Detector HDL Optimized/4 -> Logical Operator12/2
  begin/1 -> General CRC Syndrome Detector HDL Optimized/2
  last/1 -> General CRC Syndrome Detector HDL Optimized/3
  Extract Bits1/1 -> Data Type Conversion4/1
  Extract Bits/1 -> Data Type Conversion1/1
  General CRC Syndrome Detector HDL Optimized/1 -> Terminator2/1
  Data Type Conversion/1 -> General CRC Syndrome Detector HDL Optimized/1
  data/1 -> Extract Bits1/1, Extract Bits/1
  Data Type Conversion1/1 -> Gain/1
  Sum/1 -> Data Type Conversion/1
  Gain/1 -> Sum/1
  Data Type Conversion4/1 -> Sum/2

== system rev0BB/receiver/slow_rx_baseband_outer/slow_rx_baseband_enabled/slow_rx_baseband/CoarseCFO_est ==
  note: NCO Inc Est
  note: CFO Est
  note: 4 delays
  note: 12 delays
  corr : Inport
  peak : Inport  Port=2
  stop : Inport  Port=3
  reset : Inport  Port=4  OutDataTypeStr=boolean
  Complex to Real-Imag1 : ComplexToRealImag  Commented=on
  Complex to Real-Imag2 : ComplexToRealImag  Commented=on
  Complex to Real-Imag4 : ComplexToRealImag
  Constant : Constant  Value=0  OutDataTypeStr=Inherit: Inherit via back propagation  SampleTime=-1
  Data Type Conversion : DataTypeConversion  OutDataTypeStr=single
  Data Type Conversion{3..6} (4 alike) : DataTypeConversion  Commented=on
  Delay : Delay  DelayLength=1  InitialCondition=0
  Display{1..8} (8 alike) : Display  Commented=on
  Inv 1-D Lookup Table : Lookup_n-D  Commented=on  NumberOfTableDimensions=1  BreakpointsForDimension1=[0:(x_STFRepCount+1)]  IndexSearchMethod=Evenly spaced points  Table=cat(2, [1], 1./[1:(x_STFRepCount+1)] )  InterpMethod=Flat  DiagnosticForOutOfRangeInput=Error  InternalRulePriority=Speed  OutDataTypeStr=Inherit: Inherit via back propagation  RndMeth=Simplest  InputSameDT=on
  Math Function : Math  Operator=reciprocal  SaturateOnIntegerOverflow=on
  Sum : Sum  Inputs=++|  OutDataTypeStr=Inherit: Same as first input
  Sum1 : Sum  Commented=on  Inputs=|+-
  Switch : Switch  Criteria=u2 > Threshold
  Switch1 : Switch  Criteria=u2 > Threshold
  Trigonometric Function : Trigonometry  Operator=atan2
  Trigonometric Function1 : Trigonometry  Commented=on  Operator=atan2
  Trigonometric Function2 : Trigonometry  Commented=on  Operator=atan2
  atan : Subsystem  Commented=on  AncestorBlock=helperLib/atan2
  cfo_est_control : Stateflow chart  TreatAsAtomicUnit=on
  complex_conj : helperLib/complex_conj
  complex_mult_pipelined1 : Subsystem  AncestorBlock=helperLib/complex_mult_pipelined
  pipeline_delay35 : Delay  DelayLength=regular_pipeline
  pipeline_delay_match : Delay  DelayLength=(regular_pipeline*2 + cr_mult_pipeline*2) +(regular_pipeline)
  pipeline_delay_match1 : Delay  DelayLength=(regular_pipeline*2 + cr_mult_pipeline*2) +(regular_pipeline)+(regular_pipeline)
  pipelined_gain : helperLib/pipelined_gain  g=-2^22/(2*pi*golay_type)  d=regular_pipeline
  pipelined_mult : helperLib/pipelined_mult  d=cr_mult_pipeline
  correct_step : Outport
  buffer : Outport  Port=2
  wires:
  complex_mult_pipelined1/1(Out1) -> Display3/1, Complex to Real-Imag4/1
  pipeline_delay35/1 -> Sum/1, Display7/1
  reset/1 -> Switch/2, cfo_est_control/4(rst)
  Sum/1 -> Switch1/1
  cfo_est_control/1(cur) -> Complex to Real-Imag1/1, Display4/1, complex_mult_pipelined1/1(In1)
  complex_conj/1 -> complex_mult_pipelined1/2(In2)
  cfo_est_control/2(prev) -> complex_conj/1, Complex to Real-Imag2/1, Display5/1
  cfo_est_control/4(peakCount) -> pipeline_delay_match1/1
  Math Function/1 -> pipelined_mult/2
  Switch/1 -> Delay/1
  Switch1/1 -> Switch/3
  Constant/1 -> Switch/1
  cfo_est_control/3(calcDiff) -> pipeline_delay_match/1
  pipeline_delay_match/1 -> Switch1/2
  pipeline_delay_match1/1 -> Math Function/1
  Data Type Conversion3/1 -> Trigonometric Function1/1
  Data Type Conversion4/1 -> Trigonometric Function1/2
  Complex to Real-Imag1/2 -> Data Type Conversion3/1
  Complex to Real-Imag1/1 -> Data Type Conversion4/1
  Trigonometric Function1/1 -> Sum1/1, Display2/1
  Data Type Conversion5/1 -> Trigonometric Function2/1
  Data Type Conversion6/1 -> Trigonometric Function2/2
  Complex to Real-Imag2/2 -> Data Type Conversion5/1
  Complex to Real-Imag2/1 -> Data Type Conversion6/1
  Trigonometric Function2/1 -> Sum1/2, Display1/1
  Sum1/1 -> Display6/1
  stop/1 -> cfo_est_control/3(stp)
  peak/1 -> cfo_est_control/1(peak)
  corr/1 -> cfo_est_control/2(correlation)
  cfo_est_control/5(buffer) -> buffer/1
  Complex to Real-Imag4/2 -> Trigonometric Function/1
  Complex to Real-Imag4/1 -> Trigonometric Function/2
  Trigonometric Function/1 -> pipeline_delay35/1
  Delay/1 -> Display8/1, pipelined_mult/1, Sum/2, Switch1/3
  pipelined_gain/1 -> correct_step/1
  Data Type Conversion/1 -> pipelined_gain/1
  pipelined_mult/1 -> Data Type Conversion/1

== system rev0BB/receiver/slow_rx_baseband_outer/slow_rx_baseband_enabled/slow_rx_baseband/EQ ==
  signal : Inport
  expected : Inport  Port=2
  rst : Inport  Port=3
  adapt : Inport  Port=4
  step_ff : Inport  Port=5
  step_meta_ff : Inport  Port=6
  Delay : Delay  DelayLength=1  InitialCondition=0
  Display : Display  Commented=on
  Display1 : Display  Commented=on
  Display2 : Display  Commented=on
  Sum : Sum  Inputs=++|  OutDataTypeStr=Inherit: Same as first input
  Switch : Switch  Criteria=u2 > Threshold
  lms : Subsystem  AncestorBlock=helperLib/lms
  out : Outport
  err_ff : Outport  Port=2
  weights_ff : Outport  Port=3
  wires:
  adapt/1 -> Switch/2, lms/4(adapt)
  lms/3(weights) -> weights_ff/1
  step_ff/1 -> Switch/3, Display/1
  signal/1 -> lms/1(in)
  rst/1 -> lms/3(reset)
  expected/1 -> lms/2(expected)
  lms/2(err) -> err_ff/1
  lms/1(out) -> out/1
  Switch/1 -> Delay/1
  step_meta_ff/1 -> Display1/1, Sum/1
  Delay/1 -> Display2/1, lms/5(step), Sum/2
  Sum/1 -> Switch/1

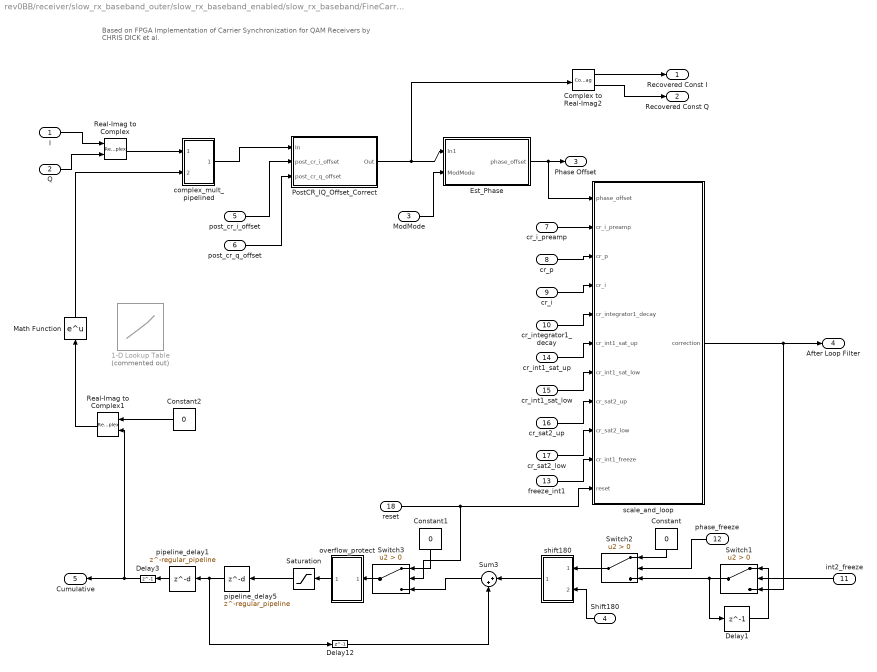
== system rev0BB/receiver/slow_rx_baseband_outer/slow_rx_baseband_enabled/slow_rx_baseband/FineCarrierRecovery ==
  note: Based on FPGA Implementation of Carrier Synchronization for QAM Receivers
      | by CHRIS DICK et al.
  I : Inport  PortDimensions=1
  Q : Inport  Port=2  PortDimensions=1
  ModMode : Inport  Port=3  PortDimensions=1
  Shift180 : Inport  Port=4  OutDataTypeStr=boolean  PortDimensions=1
  post_cr_i_offset : Inport  Port=5
  post_cr_q_offset : Inport  Port=6
  cr_i_preamp : Inport  Port=7
  cr_p : Inport  Port=8
  cr_i : Inport  Port=9
  cr_integrator1_decay : Inport  Port=10
  int2_freeze : Inport  Port=11  OutDataTypeStr=boolean
  phase_freeze : Inport  Port=12  OutDataTypeStr=boolean
  freeze_int1 : Inport  Port=13
  cr_int1_sat_up : Inport  Port=14
  cr_int1_sat_low : Inport  Port=15
  cr_sat2_up : Inport  Port=16
  cr_sat2_low : Inport  Port=17
  reset : Inport  Port=18
  1-D Lookup Table : Lookup_n-D  Commented=on  NumberOfTableDimensions=1  BreakpointsForDimension1=[-expDomain:expResolution:expDomain]  IndexSearchMethod=Evenly spaced points  Table=exp(i*[-expDomain:expResolution:expDomain])  InterpMethod=Flat  DiagnosticForOutOfRangeInput=Error  InternalRulePriority=Speed  RndMeth=Simplest  InputSameDT=on
  Complex to Real-Imag2 : ComplexToRealImag
  Constant : Constant  Value=0  OutDataTypeStr=Inherit: Inherit via back propagation  SampleTime=-1
  Constant1 : Constant  Value=0  OutDataTypeStr=Inherit: Inherit via back propagation  SampleTime=-1
  Constant2 : Constant  Value=0  OutDataTypeStr=Inherit: Inherit via back propagation
  Delay1 : Delay  DelayLength=1  InitialCondition=0
  Delay12 : Delay  DelayLength=1
  Delay3 : Delay  DelayLength=1
  Est_Phase : Subsystem
  Math Function : Math  SaturateOnIntegerOverflow=on
  PostCR_IQ_Offset_Correct : Subsystem
  Real-Imag to Complex : RealImagToComplex
  Real-Imag to Complex1 : RealImagToComplex
  Saturation : Saturate  UpperLimit=expDomain  LowerLimit=-expDomain
  Sum3 : Sum  Inputs=|++  OutDataTypeStr=Inherit: Same as first input
  Switch1 : Switch  Criteria=u2 > Threshold
  Switch2 : Switch  Criteria=u2 > Threshold
  Switch3 : Switch  Criteria=u2 > Threshold
  complex_mult_pipelined : Subsystem  AncestorBlock=helperLib/complex_mult_pipelined
  overflow_protect : Subsystem
  pipeline_delay1 : Delay  DelayLength=regular_pipeline
  pipeline_delay5 : Delay  DelayLength=regular_pipeline
  scale_and_loop : Subsystem
  shift180 : Subsystem
  Recovered Const I : Outport  PortDimensions=1
  Recovered Const Q : Outport  Port=2  PortDimensions=1
  Phase Offset : Outport  Port=3  PortDimensions=1
  After Loop Filter : Outport  Port=4  PortDimensions=1
  Cumulative : Outport  Port=5  PortDimensions=1
  wires:
  I/1 -> Real-Imag to Complex/1
  Q/1 -> Real-Imag to Complex/2
  shift180/1(Out1) -> Sum3/1
  Math Function/1 -> complex_mult_pipelined/2(In2)
  Real-Imag to Complex/1 -> complex_mult_pipelined/1(In1)
  Complex to Real-Imag2/1 -> Recovered Const I/1
  Complex to Real-Imag2/2 -> Recovered Const Q/1
  Est_Phase/1(phase_offset) -> scale_and_loop/1(phase_offset), Phase Offset/1
  overflow_protect/1(Out1) -> Saturation/1
  Shift180/1 -> shift180/2(shift180)
  scale_and_loop/1(correction) -> After Loop Filter/1, Switch1/3
  pipeline_delay1/1 -> Delay3/1
  PostCR_IQ_Offset_Correct/1(Out) -> Complex to Real-Imag2/1, Est_Phase/1(In1)
  complex_mult_pipelined/1(Out1) -> PostCR_IQ_Offset_Correct/1(In)
  post_cr_i_offset/1 -> PostCR_IQ_Offset_Correct/2(post_cr_i_offset)
  post_cr_q_offset/1 -> PostCR_IQ_Offset_Correct/3(post_cr_q_offset)
  cr_i_preamp/1 -> scale_and_loop/2(cr_i_preamp)
  cr_p/1 -> scale_and_loop/3(cr_p)
  cr_i/1 -> scale_and_loop/4(cr_i)
  cr_integrator1_decay/1 -> scale_and_loop/5(cr_integrator1_decay)
  Delay1/1 -> Switch1/1
  int2_freeze/1 -> Switch1/2
  Switch1/1 -> Switch2/3, Delay1/1
  pipeline_delay5/1 -> Delay12/1, pipeline_delay1/1
  cr_int1_sat_up/1 -> scale_and_loop/6(cr_int1_sat_up)
  cr_int1_sat_low/1 -> scale_and_loop/7(cr_int1_sat_low)
  cr_sat2_up/1 -> scale_and_loop/8(cr_sat2_up)
  cr_sat2_low/1 -> scale_and_loop/9(cr_sat2_low)
  phase_freeze/1 -> Switch2/2
  Constant/1 -> Switch2/1
  freeze_int1/1 -> scale_and_loop/10(cr_int1_freeze)
  Switch2/1 -> shift180/1(In1)
  Saturation/1 -> pipeline_delay5/1
  ModMode/1 -> Est_Phase/2(ModMode)
  Switch3/1 -> overflow_protect/1(In1)
  Sum3/1 -> Switch3/3
  Constant1/1 -> Switch3/1
  reset/1 -> Switch3/2, scale_and_loop/11(reset)
  Constant2/1 -> Real-Imag to Complex1/1
  Delay12/1 -> Sum3/2
  Real-Imag to Complex1/1 -> Math Function/1
  Delay3/1 -> Real-Imag to Complex1/2, Cumulative/1

== system rev0BB/receiver/slow_rx_baseband_outer/slow_rx_baseband_enabled/slow_rx_baseband/Golay Correlator 32 ==
  In : Inport
  GolayCoralatorBase_fp : golayLib/GolayCoralatorBase_fp  dSub=D_32(1)  wSub=W_32(1)  mult=0
  GolayCoralatorBase_fp1 : golayLib/GolayCoralatorBase_fp  dSub=D_32(2)  wSub=W_32(2)  mult=0
  GolayCoralatorBase_fp2 : golayLib/GolayCoralatorBase_fp  dSub=D_32(3)  wSub=W_32(3)  mult=0
  GolayCoralatorBase_fp3 : golayLib/GolayCoralatorBase_fp  dSub=D_32(4)  wSub=W_32(4)  mult=0
  GolayCoralatorBase_fp4 : golayLib/GolayCoralatorBase_fp  dSub=D_32(5)  wSub=W_32(5)  mult=0
  pipeline_delay{,1..13} (14 alike) : Delay  DelayLength=regular_pipeline
  Ca : Outport
  Cb : Outport  Port=2
  wires:
  GolayCoralatorBase_fp/1 -> pipeline_delay/1
  GolayCoralatorBase_fp/2 -> pipeline_delay1/1
  GolayCoralatorBase_fp1/1 -> pipeline_delay2/1
  GolayCoralatorBase_fp1/2 -> pipeline_delay3/1
  GolayCoralatorBase_fp4/1 -> pipeline_delay8/1
  GolayCoralatorBase_fp2/1 -> pipeline_delay4/1
  GolayCoralatorBase_fp2/2 -> pipeline_delay5/1
  GolayCoralatorBase_fp3/1 -> pipeline_delay6/1
  GolayCoralatorBase_fp3/2 -> pipeline_delay7/1
  pipeline_delay9/1 -> pipeline_delay11/1
  pipeline_delay8/1 -> pipeline_delay10/1
  pipeline_delay10/1 -> pipeline_delay12/1
  In/1 -> GolayCoralatorBase_fp/2, GolayCoralatorBase_fp/1
  pipeline_delay/1 -> GolayCoralatorBase_fp1/1
  pipeline_delay1/1 -> GolayCoralatorBase_fp1/2
  pipeline_delay2/1 -> GolayCoralatorBase_fp2/1
  pipeline_delay3/1 -> GolayCoralatorBase_fp2/2
  pipeline_delay4/1 -> GolayCoralatorBase_fp3/1
  pipeline_delay6/1 -> GolayCoralatorBase_fp4/1
  pipeline_delay12/1 -> Ca/1
  pipeline_delay13/1 -> Cb/1
  pipeline_delay5/1 -> GolayCoralatorBase_fp3/2
  pipeline_delay7/1 -> GolayCoralatorBase_fp4/2
  GolayCoralatorBase_fp4/2 -> pipeline_delay9/1
  pipeline_delay11/1 -> pipeline_delay13/1
